simulink model "DigitalModulation_FSK"  (R2023b)
settings: Solver=VariableStepAuto  StartTime=0.0  StopTime=10.0  RelTol=1e-3
settings Model: Creator=Aman Tripathi  LastModifiedBy=Spedrik Webster

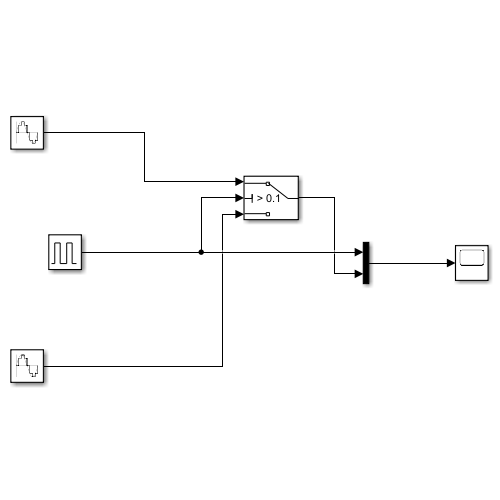
[thumbnail: Simulink's stored preview of the top-level diagram]
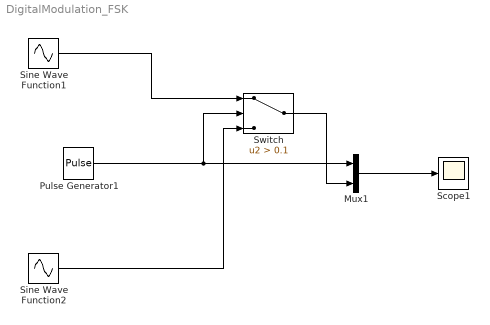
== system DigitalModulation_FSK ==
  Mux1 : Mux  Inputs=2
  Pulse Generator1 : DiscretePulseGenerator  PulseType=Time based  PulseWidth=50
  Scope1 : Scope
  Sine Wave Function1 : Sin  Frequency=20  SampleTime=1/5000
  Sine Wave Function2 : Sin  Frequency=130  SampleTime=1/5000
  Switch : Switch  Criteria=u2 > Threshold  Threshold=0.1  SaturateOnIntegerOverflow=off  InputSameDT=off
  wires:
  Mux1/1 -> Scope1/1
  Sine Wave Function2/1 -> Switch/3
  Sine Wave Function1/1 -> Switch/1
  Switch/1 -> Mux1/2
  Pulse Generator1/1 -> Mux1/1, Switch/2
